simulink library "eci_to_body"  (R2016b)
settings: Solver=VariableStepAuto  StartTime=0.0  StopTime=10.0  RelTol=1e-3
libraries: aerolibutil x1
settings Model: Creator=bbarz_000  LastModifiedBy=taylorreynolds
settings OptimizationCC: LifeSpan=inf
settings DebuggingCC: SFExecutionAtInitializationDiag=none

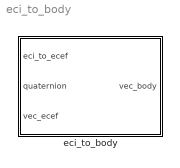
== system eci_to_body ==
  eci_to_body : Subsystem

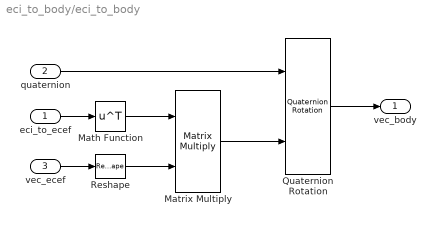
== system eci_to_body/eci_to_body ==
  eci_to_ecef : Inport
  quaternion : Inport  Port=2
  vec_ecef : Inport  Port=3
  Math Function : Math  Operator=transpose  SaturateOnIntegerOverflow=on
  Matrix Multiply : Product  Multiplication=Matrix(*)
  Quaternion Rotation : aerolibutil/Quaternion Rotation
  Reshape : Reshape  OutputDimensionality=Column vector (2-D)
  vec_body : Outport
  wires:
  vec_ecef/1 -> Reshape/1
  Math Function/1 -> Matrix Multiply/1
  quaternion/1 -> Quaternion Rotation/1
  eci_to_ecef/1 -> Math Function/1
  Matrix Multiply/1 -> Quaternion Rotation/2
  Reshape/1 -> Matrix Multiply/2
  Quaternion Rotation/1 -> vec_body/1
